simulink model "TESTE_Comunicacao_MCU"  (R2023b)
settings: Solver=VariableStepAuto  StartTime=0.0  StopTime=1  RelTol=1e-3
settings Model: Creator=Ricardo  LastModifiedBy=Ricardo

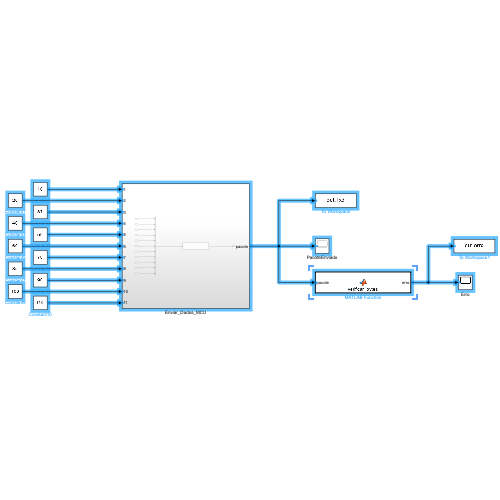
[thumbnail: Simulink's stored preview of the top-level diagram]
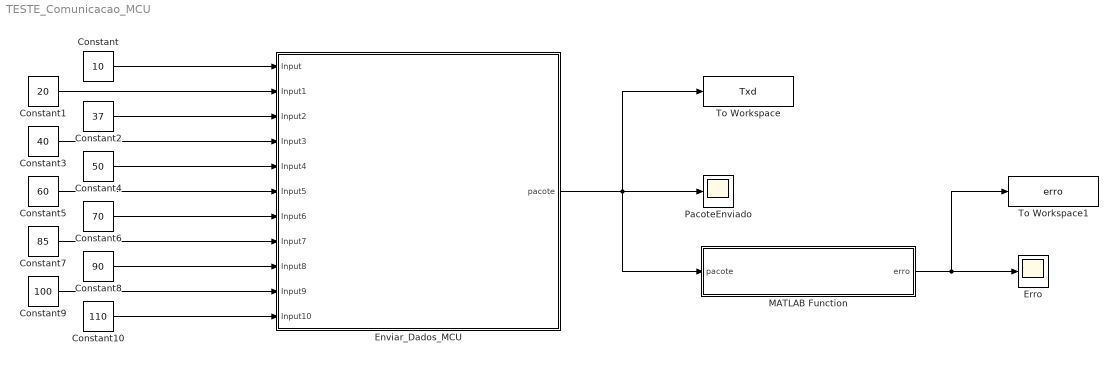
== system TESTE_Comunicacao_MCU ==
  Constant : Constant  Value=10
  Constant1 : Constant  Value=20
  Constant10 : Constant  Value=110
  Constant2 : Constant  Value=37
  Constant3 : Constant  Value=40
  Constant4 : Constant  Value=50
  Constant5 : Constant  Value=60
  Constant6 : Constant  Value=70
  Constant7 : Constant  Value=85
  Constant8 : Constant  Value=90
  Constant9 : Constant  Value=100
  Enviar_Dados_MCU : Subsystem
  Erro : Scope
  MATLAB Function : MATLAB Function  TreatAsAtomicUnit=on
  PacoteEnviado : Scope
  To Workspace : ToWorkspace  VariableName=Txd  SaveFormat=Timeseries  SampleTime=-1
  To Workspace1 : ToWorkspace  VariableName=erro  SaveFormat=Timeseries  SampleTime=-1
  wires:
  Constant/1 -> Enviar_Dados_MCU/1(Input)
  Constant1/1 -> Enviar_Dados_MCU/2(Input1)
  Constant2/1 -> Enviar_Dados_MCU/3(Input2)
  Constant3/1 -> Enviar_Dados_MCU/4(Input3)
  Constant4/1 -> Enviar_Dados_MCU/5(Input4)
  Constant6/1 -> Enviar_Dados_MCU/7(Input6)
  Constant5/1 -> Enviar_Dados_MCU/6(Input5)
  Constant7/1 -> Enviar_Dados_MCU/8(Input7)
  Constant8/1 -> Enviar_Dados_MCU/9(Input8)
  Constant10/1 -> Enviar_Dados_MCU/11(Input10)
  Constant9/1 -> Enviar_Dados_MCU/10(Input9)
  Enviar_Dados_MCU/1(pacote) -> MATLAB Function/1(pacote), To Workspace/1, PacoteEnviado/1
  MATLAB Function/1(erro) -> To Workspace1/1, Erro/1

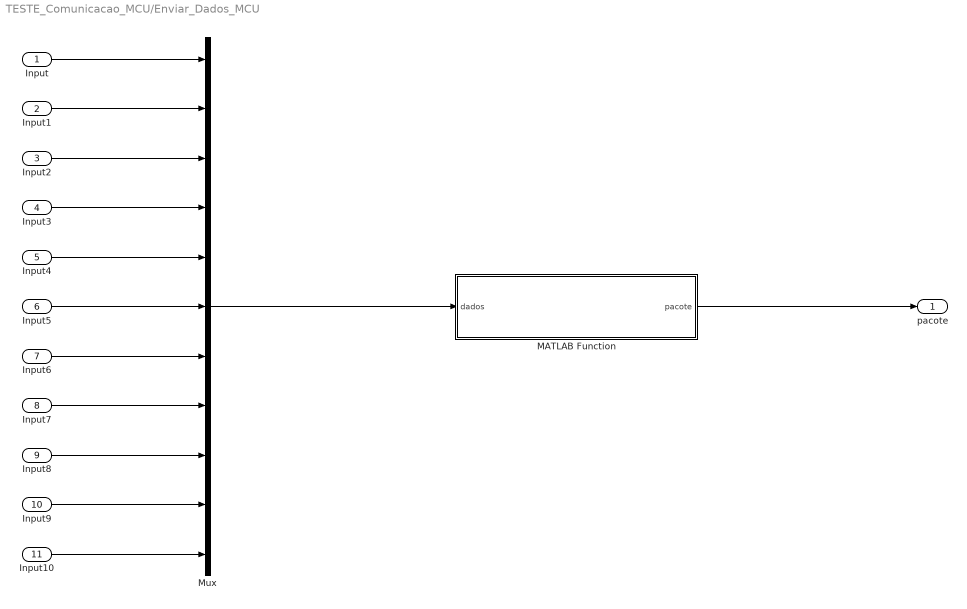
== system TESTE_Comunicacao_MCU/Enviar_Dados_MCU ==
  Input : Inport
  Input1 : Inport  Port=2
  Input2 : Inport  Port=3
  Input3 : Inport  Port=4
  Input4 : Inport  Port=5
  Input5 : Inport  Port=6
  Input6 : Inport  Port=7
  Input7 : Inport  Port=8
  Input8 : Inport  Port=9
  Input9 : Inport  Port=10
  Input10 : Inport  Port=11
  MATLAB Function : MATLAB Function  TreatAsAtomicUnit=on
  Mux : Mux  Inputs=11
  pacote : Outport
  wires:
  Input10/1 -> Mux/11
  Mux/1 -> MATLAB Function/1(dados)
  MATLAB Function/1(pacote) -> pacote/1
  Input7/1 -> Mux/8
  Input/1 -> Mux/1
  Input9/1 -> Mux/10
  Input4/1 -> Mux/5
  Input8/1 -> Mux/9
  Input2/1 -> Mux/3
  Input1/1 -> Mux/2
  Input5/1 -> Mux/6
  Input6/1 -> Mux/7
  Input3/1 -> Mux/4

== matlab function TESTE_Comunicacao_MCU/Enviar_Dados_MCU/MATLAB Function ==
  data: dados input; pacote output
function pacote = montar_pacote(dados)
    START_BYTE = uint8(170); % 0xAA
    PACKET_TYPE = uint8(1);  % 0x01 para entrada
    END_BYTE = uint8(85);    % 0x55

    % Garante que dados seja um vetor coluna de 11 elementos
    dados = reshape(dados, [], 1);
    if length(dados) ~= 11
        error('Número incorreto de entradas. Esperado: 11');
    end

    % Converte dados para bytes
    dados_bytes = typecast(dados, 'uint8');
    comprimento = uint8(length(dados_bytes));

    % Verifica se o comprimento dos dados_bytes é 88 (11*8)
    if comprimento ~= 88
        error('Comprimento dos dados bytes incorreto. Esperado: 88');
    end

    % Pré-aloca o pacote com o tamanho correto (93 bytes)
    pacote = zeros(93, 1, 'uint8');

    % Monta o pacote
    pacote(1) = START_BYTE;
    pacote(2) = PACKET_TYPE;
    pacote(3) = comprimento;
    pacote(4:4+length(dados_bytes)-1) = dados_bytes;

    % Calcula e adiciona o checksum
    checksum = uint8(mod(sum(pacote(2:end-2)), 256));
    pacote(end-1) = checksum;
    pacote(end) = END_BYTE;
end

== matlab function TESTE_Comunicacao_MCU/MATLAB Function ==
  data: pacote input; erro output
function erro = verificar_bytes(pacote)
    % Inicializa a variável de erro
    erro = 0;
    
    % Tamanho esperado do pacote
    tamanho_pacote_esperado = 93; % Pacote completo esperado

    % Verifica e imprime o tamanho do pacote recebido
    tamanho_pacote_recebido = length(pacote);
    disp(['Tamanho do pacote recebido: ', sprintf('%d', int32(tamanho_pacote_recebido))]);
    
    if tamanho_pacote_recebido ~= tamanho_pacote_esperado
        disp('Erro: Tamanho do pacote incorreto.');
        erro = 1;
        return;
    end
    
    % Inicializa variáveis para a tabela
    valores = zeros(11, 1);
    valores_esperados = (1:11)' * 10;

    % Analisa cada valor no pacote (excluindo os bytes de controle)
    for i = 1:11
        start_index = 4 + (i-1)*8;
        bytes = pacote(start_index:start_index+7);
        valor = typecast(uint8(bytes), 'double');
        valores(i) = valor;
        
        % Verifica se o valor é o esperado (por exemplo, 10, 20, ..., 110)
        valor_esperado = valores_esperados(i);
        if valor ~= valor_esperado
            disp(['Erro: Valor ', sprintf('%d', int32(i)), ' incorreto. Esperado: ', sprintf('%d', int32(valor_esperado)), ', Recebido: ', sprintf('%f', valor)]);
            erro = 1;
        end
    end
    
    % Imprimir os valores em formato de array
    disp('Índice   Esperado   Recebido');
    for i = 1:11
        disp([sprintf('%d', int32(i)), '         ', sprintf('%d', int32(valores_esperados(i))), '         ', sprintf('%f', valores(i))]);
    end
    
    if erro == 0
        disp('Todos os valores estão corretos.');
    end
end
